simulink model "kalman_sim_2020a"  (R2020a)
settings: Solver=VariableStepAuto  StartTime=0.0  StopTime=15  RelTol=1e-3
InitFcn:
  | A = diag([-1,-2,-3]);
  | B = [1;-1;1];
  | C = [0,1,0];
  | D = 0;
  | DISC = c2d(ss(A,B,C,D),0.01);
  | A = DISC.a;
  | B = DISC.b;
undefined symbols (not defined in the file or in its folder): Discrete, Time
libraries: simulink x2, ctrlSharedLib x1
settings Model: Creator=ildeberto  LastModifiedBy=idlsa
settings DebuggingCC: UnconnectedInputMsg=none  UnconnectedOutputMsg=none  UnconnectedLineMsg=none
settings ModelReferenceCC: EnableRefExpFcnMdlSchedulingChecks=off
settings RTWCC: Description=Generic Real-Time Target

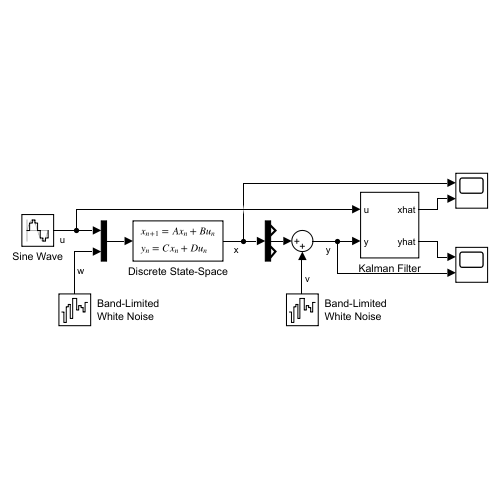
[thumbnail: Simulink's stored preview of the top-level diagram]
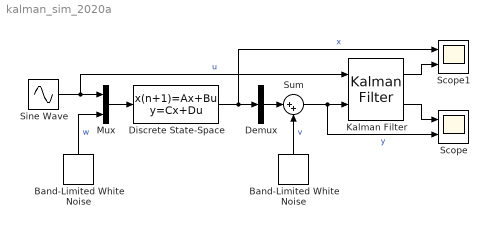
== system kalman_sim_2020a ==
  Band-Limited White Noise : simulink/Sources/Band-Limited White Noise  Cov=[0.01]  Ts=0.01  seed=[23341]
  "Band-Limited White Noise " : simulink/Sources/Band-Limited White Noise  Cov=[1e-4;1e-4;1e-4]*1  Ts=0.01  seed=[23341]
  Demux : Demux  Outputs=3
  Discrete State-Space : DiscreteStateSpace  A=A  B=[B eye(3)]  C=eye(3)  D=zeros(3,4)  SampleTime=0.01
  Kalman Filter : ctrlSharedLib/Kalman Filter  TimeDomain=Discrete-Time  UseCurrentEstimator=on  ModelSource=LTI State-Space Variable  ModelSourceVariable=ss(A,B,C,D,0.01)  A=0.95  B=1  C=1  D=0  NumberOfStates=1  NumberOfInputs=1  NumberOfOutputs=1  InitialEstimateSource=Dialog  X0=[0.3;0.6;0.9]  P0=10  UseK=off  UseGH=off  NumberOfProcessNoiseInputs=1  G=1  TimeInvariantG=on  H=0  TimeInvariantH=on  Q=0.01  TimeInvariantQ=on  R=100  TimeInvariantR=on  N=0  TimeInvariantN=on  AddInputPort=on  AddEnablePort=off  OutputEstimatedY=on  OutputP=off  Ts=-1
  Mux : Mux  Inputs=2
  Scope : Scope  NumInputPorts=2
  Scope1 : Scope  NumInputPorts=2
  Sine Wave : Sin  Amplitude=5  SampleTime=0.01
  Sum : Sum  Inputs=|++
  wires:
  Discrete State-Space/1 -> Scope1/1, Demux/1  "x"
  Band-Limited White Noise/1 -> Sum/2  "v"
  Sum/1 -> Scope/2, Kalman Filter/2  "y"
  Kalman Filter/2 -> Scope/1
  Kalman Filter/1 -> Scope1/2
  Demux/2 -> Sum/1
  Sine Wave/1 -> Kalman Filter/1, Mux/1  "u"
  "Band-Limited White Noise "/1 -> Mux/2  "w"
  Mux/1 -> Discrete State-Space/1
